simulink model "zad7_sim"  (R2022b)
settings: Solver=VariableStepAuto  StartTime=0.0  StopTime=3  RelTol=1e-3
values from neighbouring files (symbols this model uses):
  k1 = K(1)    [zad3.m]    (also in zadanie_dodatkowe.m)
  k2 = K(2)    [zad3.m]    (also in zadanie_dodatkowe.m)
  k3 = K(3)    [zad3.m]    (also in zadanie_dodatkowe.m)
  l1 = L(1)    [zad4.m]
  l2 = L(2)    [zad4.m]
  l3 = L(3)    [zad4.m]
settings Model: Creator=Mat  LastModifiedBy=Mat

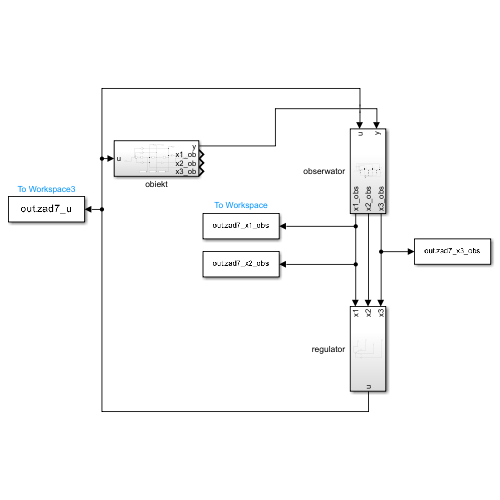
[thumbnail: Simulink's stored preview of the top-level diagram]
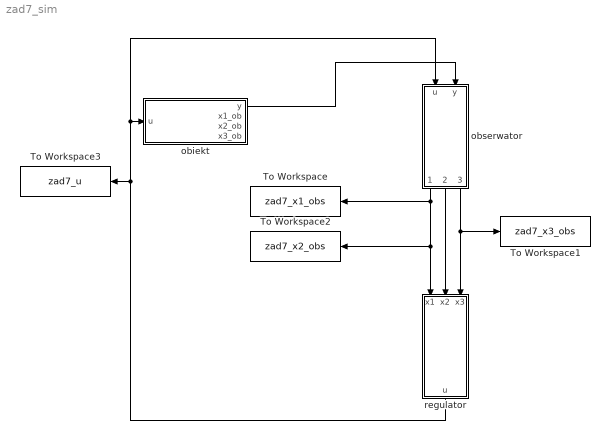
== system zad7_sim ==
  To Workspace : ToWorkspace  VariableName=zad7_x1_obs  SaveFormat=Timeseries  SampleTime=-1
  To Workspace1 : ToWorkspace  VariableName=zad7_x3_obs  SaveFormat=Timeseries  SampleTime=-1
  To Workspace2 : ToWorkspace  VariableName=zad7_x2_obs  SaveFormat=Timeseries  SampleTime=-1
  To Workspace3 : ToWorkspace  VariableName=zad7_u  SaveFormat=Timeseries  SampleTime=-1
  obiekt : Subsystem
  obserwator : Subsystem
  regulator : Subsystem
  wires:
  regulator/1(u) -> To Workspace3/1, obserwator/1(u), obiekt/1(u)
  obiekt/1(y) -> obserwator/2(y)
  obserwator/1(x1_obs) -> To Workspace/1, To Workspace2/1, regulator/1(x1)
  obserwator/2(x2_obs) -> regulator/2(x2)
  obserwator/3(x3_obs) -> To Workspace1/1, regulator/3(x3)

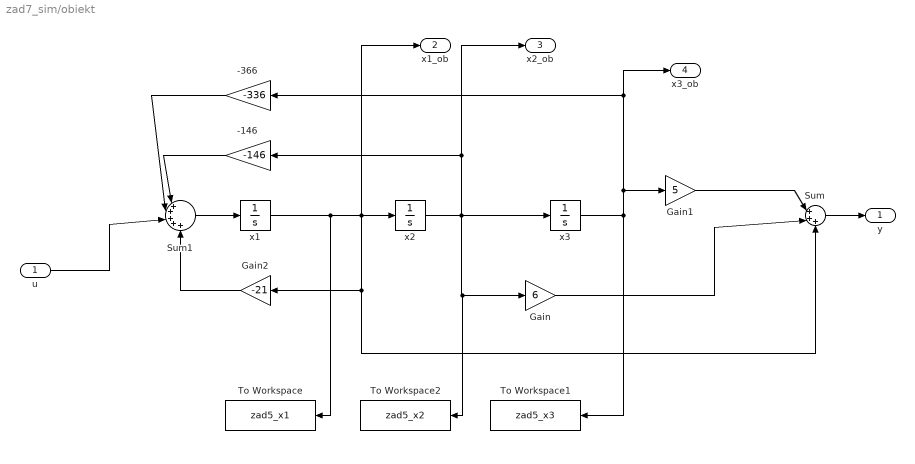
== system zad7_sim/obiekt ==
  u : Inport
  -146 : Gain  Gain=-146
  -366 : Gain  Gain=-336
  Gain : Gain  Gain=6
  Gain1 : Gain  Gain=5
  Gain2 : Gain  Gain=-21
  Sum : Sum  Inputs=|+++
  Sum1 : Sum  Inputs=|+++++
  To Workspace : ToWorkspace  VariableName=zad5_x1  SaveFormat=Timeseries  SampleTime=-1
  To Workspace1 : ToWorkspace  VariableName=zad5_x3  SaveFormat=Timeseries  SampleTime=-1
  To Workspace2 : ToWorkspace  VariableName=zad5_x2  SaveFormat=Timeseries  SampleTime=-1
  x1 : Integrator  InitialCondition=-1
  x2 : Integrator  InitialCondition=-2
  x3 : Integrator  InitialCondition=-3
  y : Outport
  x1_ob : Outport  Port=2
  x2_ob : Outport  Port=3
  x3_ob : Outport  Port=4
  wires:
  Gain2/1 -> Sum1/5
  -366/1 -> Sum1/2
  Gain1/1 -> Sum/1
  x3/1 -> To Workspace1/1, Gain1/1, x3_ob/1, -366/1
  x1/1 -> To Workspace/1, x1_ob/1, Gain2/1, Sum/3, x2/1
  Sum/1 -> y/1
  -146/1 -> Sum1/1
  u/1 -> Sum1/3
  x2/1 -> x2_ob/1, -146/1, x3/1, To Workspace2/1, Gain/1
  Gain/1 -> Sum/2
  Sum1/1 -> x1/1

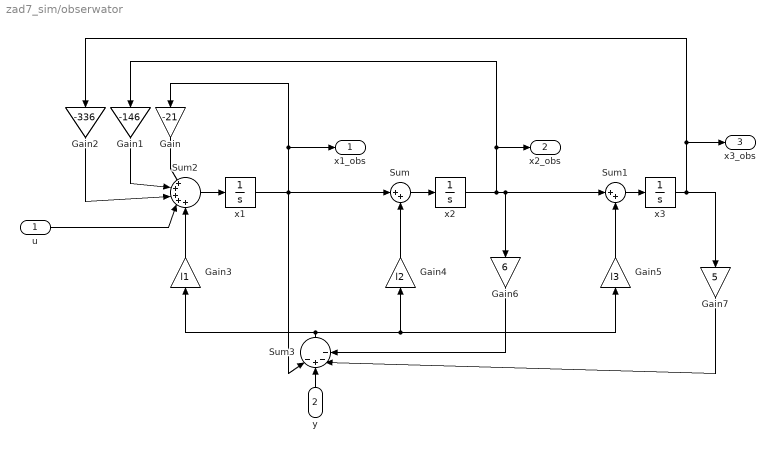
== system zad7_sim/obserwator ==
  u : Inport
  y : Inport  Port=2
  Gain : Gain  Gain=-21
  Gain1 : Gain  Gain=-146
  Gain2 : Gain  Gain=-336
  Gain3 : Gain  Gain=l1
  Gain4 : Gain  Gain=l2
  Gain5 : Gain  Gain=l3
  Gain6 : Gain  Gain=6
  Gain7 : Gain  Gain=5
  Sum : Sum  Inputs=|++
  Sum1 : Sum  Inputs=|++
  Sum2 : Sum  Inputs=|+++++
  Sum3 : Sum  Inputs=|-+--
  x1 : Integrator
  x2 : Integrator
  x3 : Integrator
  x1_obs : Outport
  x2_obs : Outport  Port=2
  x3_obs : Outport  Port=3
  wires:
  Gain4/1 -> Sum/2
  Sum1/1 -> x3/1
  x2/1 -> Gain6/1, Sum1/1, x2_obs/1, Gain1/1
  Sum3/1 -> Gain4/1, Gain5/1, Gain3/1
  Gain1/1 -> Sum2/2
  x3/1 -> Gain7/1, x3_obs/1, Gain2/1
  Gain/1 -> Sum2/1
  Gain6/1 -> Sum3/4
  x1/1 -> Sum3/1, x1_obs/1, Gain/1, Sum/1
  Gain7/1 -> Sum3/3
  Sum2/1 -> x1/1
  Gain3/1 -> Sum2/5
  Gain5/1 -> Sum1/2
  Sum/1 -> x2/1
  u/1 -> Sum2/4
  Gain2/1 -> Sum2/3
  y/1 -> Sum3/2

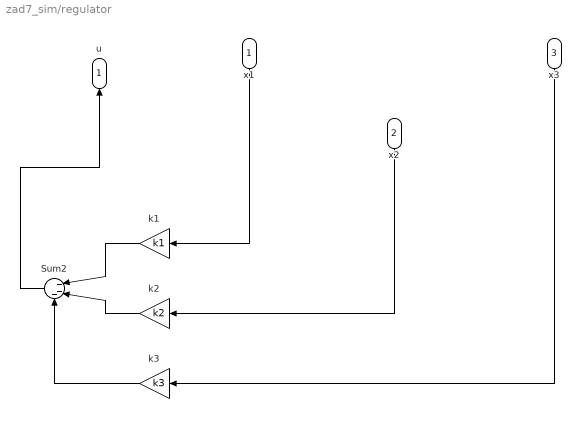
== system zad7_sim/regulator ==
  x1 : Inport
  x2 : Inport  Port=2
  x3 : Inport  Port=3
  Sum2 : Sum  Inputs=|---
  k1 : Gain  Gain=k1
  k2 : Gain  Gain=k2
  k3 : Gain  Gain=k3
  u : Outport
  wires:
  Sum2/1 -> u/1
  k2/1 -> Sum2/2
  x3/1 -> k3/1
  k3/1 -> Sum2/3
  k1/1 -> Sum2/1
  x2/1 -> k2/1
  x1/1 -> k1/1
